simulink model "z331c_Sim"  (Simulink 7.1)
settings: Solver=ode45  StartTime=-10.0  StopTime=10.0  RelTol=1e-3
settings Model: Creator=mestar  LastModifiedBy=mestar
settings DebuggingCC: SolverPrmCheckMsg=none

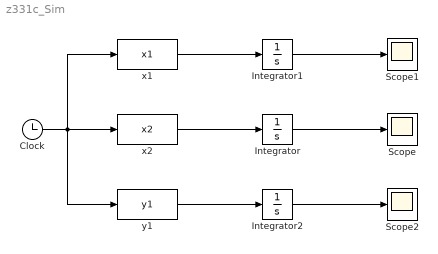
== system z331c_Sim ==
  Clock : Clock
      settings: Decimation=10
  Integrator : Integrator
  Integrator1 : Integrator
  Integrator2 : Integrator
  Scope : Scope
  Scope1 : Scope
  Scope2 : Scope
      settings: SaveName=ScopeData2
  x1 : MATLABFcn  MATLABFcn=x1
  x2 : MATLABFcn  MATLABFcn=x2
  y1 : MATLABFcn  MATLABFcn=y1
  wires:
  Clock/1 -> x2/1, y1/1, x1/1
  x2/1 -> Integrator/1
  Integrator/1 -> Scope/1
  x1/1 -> Integrator1/1
  Integrator1/1 -> Scope1/1
  y1/1 -> Integrator2/1
  Integrator2/1 -> Scope2/1
